simulink model "trajectory_gen"  (R2020a)
settings: Solver=VariableStepAuto  StartTime=0.0  StopTime=10.0  RelTol=1e-3
libraries: dsppolyfun x6, simulink x6
settings Model: Creator=nswve  LastModifiedBy=UNIST
settings DataIOCC: ReturnWorkspaceOutputs=off
settings DebuggingCC: ArithmeticOperatorsInVariantConditions=warning
settings SFSimCC: SimUseLocalCustomCode=off  CustomCodeUndefinedFunction=UseInterfaceOnly
settings RTWCC: RTWUseLocalCustomCode=off

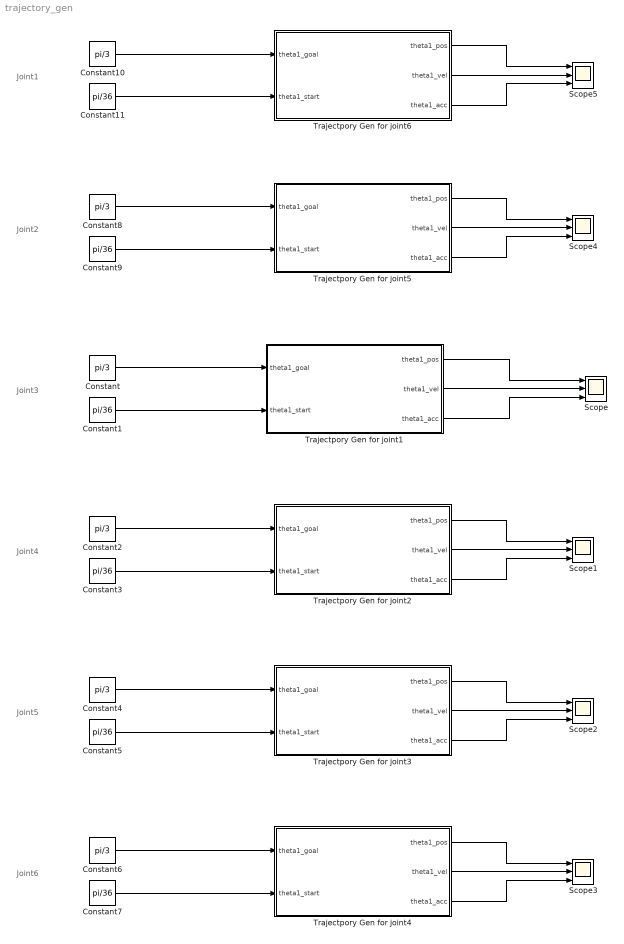
== system trajectory_gen ==
  note: Joint1
  note: Joint2
  note: Joint3
  note: Joint4
  note: Joint5
  note: Joint6
  Constant{,2,4,6,8,10} (6 alike) : Constant  Value=pi/3
  Constant{1,3,5,7,9,11} (6 alike) : Constant  Value=pi/36
  Scope{,1..5} (6 alike) : Scope  NumInputPorts=3
  Trajectpory Gen for joint1 : Subsystem
  Trajectpory Gen for joint2 : Subsystem
  Trajectpory Gen for joint3 : Subsystem
  Trajectpory Gen for joint4 : Subsystem
  Trajectpory Gen for joint5 : Subsystem
  Trajectpory Gen for joint6 : Subsystem
  wires:
  Constant/1 -> Trajectpory Gen for joint1/1("theta1_goal ")
  Constant1/1 -> Trajectpory Gen for joint1/2("theta1_start ")
  Trajectpory Gen for joint1/1("theta1_pos ") -> Scope/1
  Trajectpory Gen for joint1/2("theta1_vel ") -> Scope/2
  Trajectpory Gen for joint1/3("theta1_acc ") -> Scope/3
  Trajectpory Gen for joint2/1("theta1_pos ") -> Scope1/1
  Constant3/1 -> Trajectpory Gen for joint2/2("theta1_start ")
  Trajectpory Gen for joint2/2("theta1_vel ") -> Scope1/2
  Trajectpory Gen for joint2/3("theta1_acc ") -> Scope1/3
  Constant2/1 -> Trajectpory Gen for joint2/1("theta1_goal ")
  Constant4/1 -> Trajectpory Gen for joint3/1("theta1_goal ")
  Trajectpory Gen for joint3/2("theta1_vel ") -> Scope2/2
  Constant5/1 -> Trajectpory Gen for joint3/2("theta1_start ")
  Trajectpory Gen for joint3/1("theta1_pos ") -> Scope2/1
  Trajectpory Gen for joint3/3("theta1_acc ") -> Scope2/3
  Trajectpory Gen for joint4/3("theta1_acc ") -> Scope3/3
  Trajectpory Gen for joint4/1("theta1_pos ") -> Scope3/1
  Trajectpory Gen for joint4/2("theta1_vel ") -> Scope3/2
  Constant6/1 -> Trajectpory Gen for joint4/1("theta1_goal ")
  Constant7/1 -> Trajectpory Gen for joint4/2("theta1_start ")
  Trajectpory Gen for joint5/2("theta1_vel ") -> Scope4/2
  Trajectpory Gen for joint5/1("theta1_pos ") -> Scope4/1
  Trajectpory Gen for joint5/3("theta1_acc ") -> Scope4/3
  Constant9/1 -> Trajectpory Gen for joint5/2("theta1_start ")
  Constant8/1 -> Trajectpory Gen for joint5/1("theta1_goal ")
  Constant11/1 -> Trajectpory Gen for joint6/2("theta1_start ")
  Trajectpory Gen for joint6/1("theta1_pos ") -> Scope5/1
  Trajectpory Gen for joint6/2("theta1_vel ") -> Scope5/2
  Constant10/1 -> Trajectpory Gen for joint6/1("theta1_goal ")
  Trajectpory Gen for joint6/3("theta1_acc ") -> Scope5/3

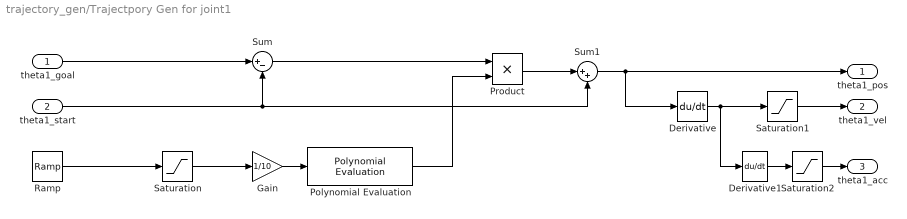
== system trajectory_gen/Trajectpory Gen for joint1 ==
  "theta1_goal " : Inport
  "theta1_start " : Inport  Port=2
  Derivative : Derivative
  Derivative1 : Derivative
  Gain : Gain  Gain=1/10
  Polynomial Evaluation : dsppolyfun/Polynomial Evaluation  useConstCoeffs=on  constCoeffs=[6 -15 10 0 0 0]
      settings: SourceProductBaseCode=DS
  Product : Product
  Ramp : simulink/Sources/Ramp  slope=1  start=0  InitialOutput=0
  Saturation : Saturate  UpperLimit=10  LowerLimit=-10
  Saturation1 : Saturate
  Saturation2 : Saturate
  Sum : Sum  Inputs=|+-
  Sum1 : Sum  Inputs=|++
  "theta1_pos " : Outport  VectorParamsAs1DForOutWhenUnconnected=off
  "theta1_vel " : Outport  Port=2  VectorParamsAs1DForOutWhenUnconnected=off
  "theta1_acc " : Outport  Port=3  VectorParamsAs1DForOutWhenUnconnected=off
  wires:
  "theta1_start "/1 -> Sum1/2, Sum/2
  Sum/1 -> Product/1
  "theta1_goal "/1 -> Sum/1
  Sum1/1 -> Derivative/1, "theta1_pos "/1
  Derivative1/1 -> Saturation2/1
  Saturation1/1 -> "theta1_vel "/1
  Gain/1 -> Polynomial Evaluation/1
  Product/1 -> Sum1/1
  Polynomial Evaluation/1 -> Product/2
  Saturation2/1 -> "theta1_acc "/1
  Saturation/1 -> Gain/1
  Ramp/1 -> Saturation/1
  Derivative/1 -> Derivative1/1, Saturation1/1

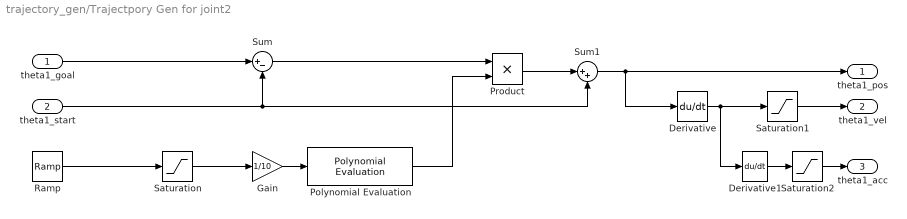
== system trajectory_gen/Trajectpory Gen for joint2 ==
  "theta1_goal " : Inport
  "theta1_start " : Inport  Port=2
  Derivative : Derivative
  Derivative1 : Derivative
  Gain : Gain  Gain=1/10
  Polynomial Evaluation : dsppolyfun/Polynomial Evaluation  useConstCoeffs=on  constCoeffs=[6 -15 10 0 0 0]
      settings: SourceProductBaseCode=DS
  Product : Product
  Ramp : simulink/Sources/Ramp  slope=1  start=0  InitialOutput=0
  Saturation : Saturate  UpperLimit=10  LowerLimit=-10
  Saturation1 : Saturate
  Saturation2 : Saturate
  Sum : Sum  Inputs=|+-
  Sum1 : Sum  Inputs=|++
  "theta1_pos " : Outport  VectorParamsAs1DForOutWhenUnconnected=off
  "theta1_vel " : Outport  Port=2  VectorParamsAs1DForOutWhenUnconnected=off
  "theta1_acc " : Outport  Port=3  VectorParamsAs1DForOutWhenUnconnected=off
  wires:
  "theta1_start "/1 -> Sum1/2, Sum/2
  Sum/1 -> Product/1
  "theta1_goal "/1 -> Sum/1
  Sum1/1 -> Derivative/1, "theta1_pos "/1
  Derivative1/1 -> Saturation2/1
  Saturation1/1 -> "theta1_vel "/1
  Gain/1 -> Polynomial Evaluation/1
  Product/1 -> Sum1/1
  Polynomial Evaluation/1 -> Product/2
  Saturation2/1 -> "theta1_acc "/1
  Saturation/1 -> Gain/1
  Ramp/1 -> Saturation/1
  Derivative/1 -> Derivative1/1, Saturation1/1

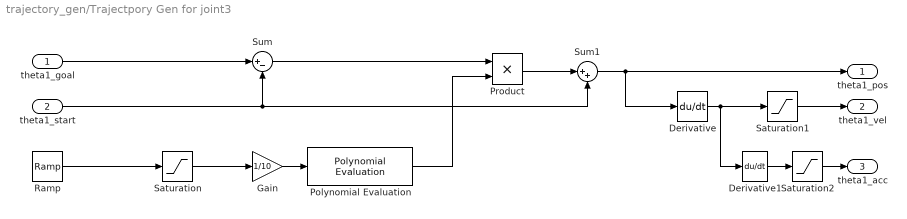
== system trajectory_gen/Trajectpory Gen for joint3 ==
  "theta1_goal " : Inport
  "theta1_start " : Inport  Port=2
  Derivative : Derivative
  Derivative1 : Derivative
  Gain : Gain  Gain=1/10
  Polynomial Evaluation : dsppolyfun/Polynomial Evaluation  useConstCoeffs=on  constCoeffs=[6 -15 10 0 0 0]
      settings: SourceProductBaseCode=DS
  Product : Product
  Ramp : simulink/Sources/Ramp  slope=1  start=0  InitialOutput=0
  Saturation : Saturate  UpperLimit=10  LowerLimit=-10
  Saturation1 : Saturate
  Saturation2 : Saturate
  Sum : Sum  Inputs=|+-
  Sum1 : Sum  Inputs=|++
  "theta1_pos " : Outport  VectorParamsAs1DForOutWhenUnconnected=off
  "theta1_vel " : Outport  Port=2  VectorParamsAs1DForOutWhenUnconnected=off
  "theta1_acc " : Outport  Port=3  VectorParamsAs1DForOutWhenUnconnected=off
  wires:
  "theta1_start "/1 -> Sum1/2, Sum/2
  Sum/1 -> Product/1
  "theta1_goal "/1 -> Sum/1
  Sum1/1 -> Derivative/1, "theta1_pos "/1
  Derivative1/1 -> Saturation2/1
  Saturation1/1 -> "theta1_vel "/1
  Gain/1 -> Polynomial Evaluation/1
  Product/1 -> Sum1/1
  Polynomial Evaluation/1 -> Product/2
  Saturation2/1 -> "theta1_acc "/1
  Saturation/1 -> Gain/1
  Ramp/1 -> Saturation/1
  Derivative/1 -> Derivative1/1, Saturation1/1

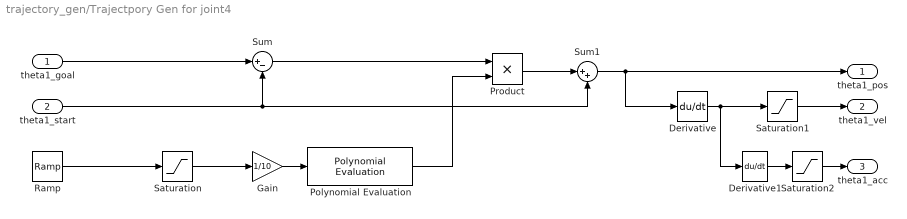
== system trajectory_gen/Trajectpory Gen for joint4 ==
  "theta1_goal " : Inport
  "theta1_start " : Inport  Port=2
  Derivative : Derivative
  Derivative1 : Derivative
  Gain : Gain  Gain=1/10
  Polynomial Evaluation : dsppolyfun/Polynomial Evaluation  useConstCoeffs=on  constCoeffs=[6 -15 10 0 0 0]
      settings: SourceProductBaseCode=DS
  Product : Product
  Ramp : simulink/Sources/Ramp  slope=1  start=0  InitialOutput=0
  Saturation : Saturate  UpperLimit=10  LowerLimit=-10
  Saturation1 : Saturate
  Saturation2 : Saturate
  Sum : Sum  Inputs=|+-
  Sum1 : Sum  Inputs=|++
  "theta1_pos " : Outport  VectorParamsAs1DForOutWhenUnconnected=off
  "theta1_vel " : Outport  Port=2  VectorParamsAs1DForOutWhenUnconnected=off
  "theta1_acc " : Outport  Port=3  VectorParamsAs1DForOutWhenUnconnected=off
  wires:
  "theta1_start "/1 -> Sum1/2, Sum/2
  Sum/1 -> Product/1
  "theta1_goal "/1 -> Sum/1
  Sum1/1 -> Derivative/1, "theta1_pos "/1
  Derivative1/1 -> Saturation2/1
  Saturation1/1 -> "theta1_vel "/1
  Gain/1 -> Polynomial Evaluation/1
  Product/1 -> Sum1/1
  Polynomial Evaluation/1 -> Product/2
  Saturation2/1 -> "theta1_acc "/1
  Saturation/1 -> Gain/1
  Ramp/1 -> Saturation/1
  Derivative/1 -> Derivative1/1, Saturation1/1

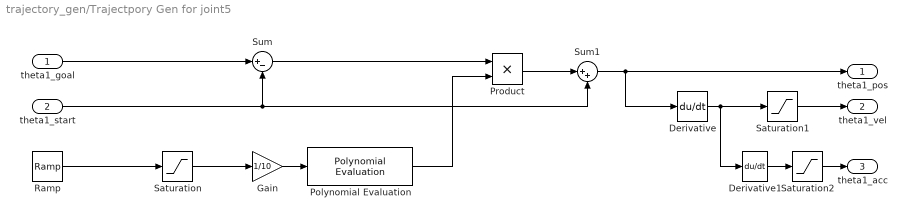
== system trajectory_gen/Trajectpory Gen for joint5 ==
  "theta1_goal " : Inport
  "theta1_start " : Inport  Port=2
  Derivative : Derivative
  Derivative1 : Derivative
  Gain : Gain  Gain=1/10
  Polynomial Evaluation : dsppolyfun/Polynomial Evaluation  useConstCoeffs=on  constCoeffs=[6 -15 10 0 0 0]
      settings: SourceProductBaseCode=DS
  Product : Product
  Ramp : simulink/Sources/Ramp  slope=1  start=0  InitialOutput=0
  Saturation : Saturate  UpperLimit=10  LowerLimit=-10
  Saturation1 : Saturate
  Saturation2 : Saturate
  Sum : Sum  Inputs=|+-
  Sum1 : Sum  Inputs=|++
  "theta1_pos " : Outport  VectorParamsAs1DForOutWhenUnconnected=off
  "theta1_vel " : Outport  Port=2  VectorParamsAs1DForOutWhenUnconnected=off
  "theta1_acc " : Outport  Port=3  VectorParamsAs1DForOutWhenUnconnected=off
  wires:
  "theta1_start "/1 -> Sum1/2, Sum/2
  Sum/1 -> Product/1
  "theta1_goal "/1 -> Sum/1
  Sum1/1 -> Derivative/1, "theta1_pos "/1
  Derivative1/1 -> Saturation2/1
  Saturation1/1 -> "theta1_vel "/1
  Gain/1 -> Polynomial Evaluation/1
  Product/1 -> Sum1/1
  Polynomial Evaluation/1 -> Product/2
  Saturation2/1 -> "theta1_acc "/1
  Saturation/1 -> Gain/1
  Ramp/1 -> Saturation/1
  Derivative/1 -> Derivative1/1, Saturation1/1

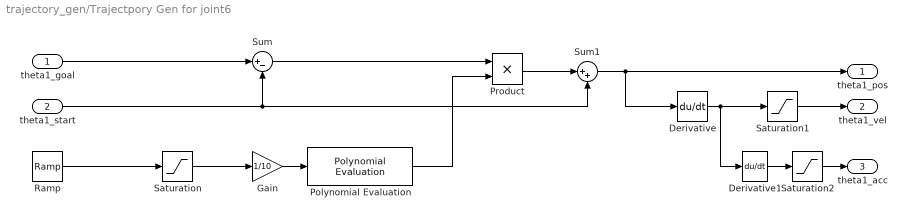
== system trajectory_gen/Trajectpory Gen for joint6 ==
  "theta1_goal " : Inport
  "theta1_start " : Inport  Port=2
  Derivative : Derivative
  Derivative1 : Derivative
  Gain : Gain  Gain=1/10
  Polynomial Evaluation : dsppolyfun/Polynomial Evaluation  useConstCoeffs=on  constCoeffs=[6 -15 10 0 0 0]
      settings: SourceProductBaseCode=DS
  Product : Product
  Ramp : simulink/Sources/Ramp  slope=1  start=0  InitialOutput=0
  Saturation : Saturate  UpperLimit=10  LowerLimit=-10
  Saturation1 : Saturate
  Saturation2 : Saturate
  Sum : Sum  Inputs=|+-
  Sum1 : Sum  Inputs=|++
  "theta1_pos " : Outport  VectorParamsAs1DForOutWhenUnconnected=off
  "theta1_vel " : Outport  Port=2  VectorParamsAs1DForOutWhenUnconnected=off
  "theta1_acc " : Outport  Port=3  VectorParamsAs1DForOutWhenUnconnected=off
  wires:
  "theta1_start "/1 -> Sum1/2, Sum/2
  Sum/1 -> Product/1
  "theta1_goal "/1 -> Sum/1
  Sum1/1 -> Derivative/1, "theta1_pos "/1
  Derivative1/1 -> Saturation2/1
  Saturation1/1 -> "theta1_vel "/1
  Gain/1 -> Polynomial Evaluation/1
  Product/1 -> Sum1/1
  Polynomial Evaluation/1 -> Product/2
  Saturation2/1 -> "theta1_acc "/1
  Saturation/1 -> Gain/1
  Ramp/1 -> Saturation/1
  Derivative/1 -> Derivative1/1, Saturation1/1
